simulink model "mdaq_vipstab"  (R2024b)
settings: Solver=FixedStepDiscrete  StartTime=0.0  StopTime=10  RelTol=1e-3  EnableMultiTasking=on
PreLoadFcn:
  | template_orig = fliplr([109 100]);
  | template_size = fliplr([18 22]);
  | search_border = fliplr([10 15]);
  | pos.template_orig = fliplr(template_orig);
  | pos.template_size = template_size;
  | pos.search_border = search_border;
  | pos.template_center = floor((template_size-1)/2);
  | pos.template_center_pos = pos.template_orig + ...
  |     pos.template_center - 1;
libraries: visionanalysis x1, visiongeotforms x1
settings Model: Tag="0  0  0  0  0  1"  CodeVerificationMode=processor-in-the-loop (pil)  Creator=The MathWorks Inc.  LastModifiedBy=benia
settings SolverCC: AlgebraicLoopSolver=TrustRegion
settings DataIOCC: LimitDataPoints=on  SaveFormat=Array  SignalLoggingSaveFormat=ModelDataLogs  SaveOutput=off  SaveTime=off  ReturnWorkspaceOutputs=off  SignalLoggingName=logsOut
settings OptimizationCC: DefaultParameterBehavior=Inlined  ExpressionDepthLimit=2147483647  InitFltsAndDblsToZero=on  LifeSpan=Inf  BufferReusableBoundary=off  EfficientTunableParamExpr=on
settings DebuggingCC: UnderspecifiedInitializationDetection=Classic  MergeDetectMultiDrivingBlocksExec=none  CheckExecutionContextPreStartOutputMsg=on  InheritedTsInSrcMsg=none  MultiTaskDSMMsg=warning  SigSpecEnsureSampleTimeMsg=none  ParameterPrecisionLossMsg=none  UnderSpecifiedDataTypeMsg=error  FcnCallInpInsideContextMsg=warning  UnconnectedInputMsg=warning  UnconnectedOutputMsg=warning  UnconnectedLineMsg=warning  BusObjectLabelMismatch=none  StateNameClashWarn=warning  SFUnexpectedBacktrackingDiag=warning  SFNoUnconditionalDefaultTransitionDiag=warning  SFExecutionAtInitializationDiag=none  ArithmeticOperatorsInVariantConditions=warning
settings HardwareCC: ProdBitPerLong=40  ProdBitPerPointer=32  ProdBitPerSizeT=32  ProdBitPerPtrDiffT=32  ProdLargestAtomicInteger=Integer  ProdLargestAtomicFloat=None  ProdWordSize=32  ProdHWDeviceType=Texas Instruments->C6000  TargetBitPerLong=64  TargetBitPerPointer=64  TargetBitPerSizeT=64  TargetBitPerPtrDiffT=64  TargetLongLongMode=on  TargetIntDivRoundTo=Zero  TargetEndianess=LittleEndian  TargetWordSize=64  TargetHWDeviceType=MATLAB Host
settings ModelReferenceCC: UpdateModelReferenceTargets=IfOutOfDate  PropagateSignalLabelsOutOfModel=off
settings SFSimCC: SimUseLocalCustomCode=off  MATLABDynamicMemAlloc=off  CustomCodeUndefinedFunction=UseInterfaceOnly
settings RTWCC: Description=MicroDAQ Real-Time Measurement System  SystemTargetFile=microdaq.tlc  TemplateMakefile=microdaq.tmf  PostCodeGenCommand=microdaq_postcodegen(buildInfo)  GenerateReport=on  RTWUseLocalCustomCode=off  IncludeHyperlinkInReport=on  GenerateCodeReplacementReport=on  GPUComputeCapability=3.5
settings CodeAppCC: IgnoreCustomStorageClasses=off  StateflowObjectComments=on
settings STFCustomTargetCC: CombineOutputUpdateFcns=on  ERTCustomFileBanners=on  SupportContinuousTime=off  SupportNonInlinedSFcns=off  RemoveResetFunc=on  MATLABClassNameForMDSCustomization=Simulink.SoftwareTarget.ERTCustomization  SystemTargetFile=microdaq.tlc
settings ERTTargetCC: MultiwordLength=2048  ParMdlRefBuildCompliant=off  CompOptLevelCompliant=off  ConcurrentExecutionCompliant=off  ModelStepFunctionPrototypeControlCompliant=off  CPPClassGenCompliant=off  UseToolchainInfoCompliant=off  ERTCustomFileTemplate=microdaq_main.tlc  ConvertIfToSwitch=off  SuppressUnreachableDefaultCases=off  DynamicArrayContainerType=coder::array
settings ConfigComp: CovMetricSettings=dw  CovSaveCumulativeToWorkspaceVar=on  CovSaveSingleToWorkspaceVar=on  CovExternalEMLEnable=off

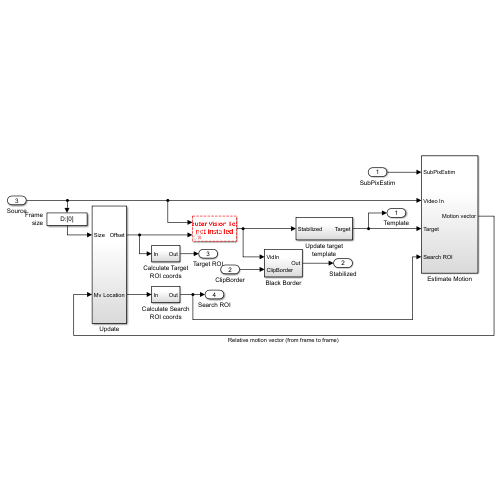
[thumbnail: Simulink's stored preview of the top-level diagram]
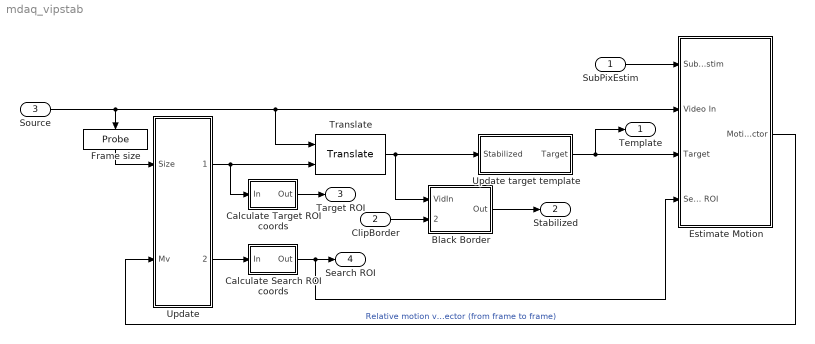
== system mdaq_vipstab ==
  SubPixEstim : Inport  OutDataTypeStr=boolean  PortDimensions=[1 1]  SampleTime=[0.033333299999999996,0]
  ClipBorder : Inport  Port=2  OutDataTypeStr=boolean  PortDimensions=[1 1]  SampleTime=[0.033333299999999996,0]
  Source : Inport  Port=3  OutDataTypeStr=uint8  PortDimensions=[320 240]  SampleTime=[0.033333299999999996,0]
  Black Border : Subsystem
  Calculate Search ROI coords : Subsystem
  Calculate Target ROI coords : Subsystem
  Estimate Motion : Subsystem
  Frame size : Probe  ProbeWidth=off  ProbeSampleTime=off  ProbeComplexSignal=off  ProbeSignalDimensions=on  ProbeDimensionsDataType=int16
  Translate : visiongeotforms/Translate  outSizeT=Same as input image  src_trans=Input port  translation="[1.5  2.3]"  maxOffset=[8 10]  fillVal=0  interpMethod=Bilinear  roundingMode=Floor  overflowMode=off  firstCoeffMode=Binary point scaling  firstCoeffWordLength=16  firstCoeffFracLength=6  prodOutputMode=Binary point scaling  prodOutputWordLength=32  prodOutputFracLength=20
  Update : Subsystem
  Update target template : Subsystem
  Template : Outport  OutDataTypeStr=uint8  PortDimensions=[22 18]  SampleTime=[0.033333299999999996,0]
  Stabilized : Outport  Port=2  OutDataTypeStr=uint8  PortDimensions=[320 240]  SampleTime=[0.033333299999999996,0]
  Target ROI : Outport  Port=3  OutDataTypeStr=fixdt('sfix16_En6')  PortDimensions=[1 4]  SampleTime=[0.033333299999999996,0]
  Search ROI : Outport  Port=4  OutDataTypeStr=fixdt('sfix16_En6')  PortDimensions=[1 4]  SampleTime=[0.033333299999999996,0]
  wires:
  Update/1(Offset) -> Calculate Target ROI coords/1(In), Translate/2
  Update/2(Location) -> Calculate Search ROI coords/1(In)
  Update target template/1(Target) -> Estimate Motion/3(Target), Template/1
  Source/1 -> Frame size/1, Estimate Motion/2(Video In), Translate/1
  Translate/1 -> Black Border/1(VidIn), Update target template/1(Stabilized)
  Estimate Motion/1(Motion vector) -> Update/2(Mv)  "Relative motion vector (from frame to frame)"
  Frame size/1 -> Update/1(Size)
  SubPixEstim/1 -> Estimate Motion/1(SubPixEstim)
  Black Border/1(Out) -> Stabilized/1
  ClipBorder/1 -> Black Border/2(ClipBorder)
  Calculate Search ROI coords/1(Out) -> Estimate Motion/4(Search ROI), Search ROI/1
  Calculate Target ROI coords/1(Out) -> Target ROI/1

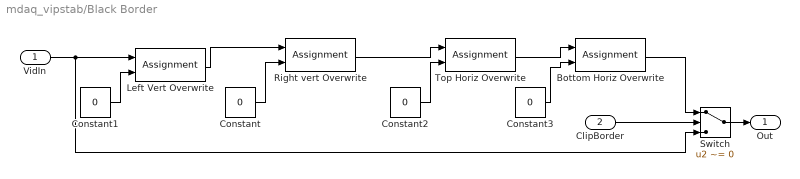
== system mdaq_vipstab/Black Border ==
  VidIn : Inport
  ClipBorder : Inport  Port=2
  Bottom Horiz Overwrite : Assignment  NumberOfDimensions=2  IndexOptions=Index vector (dialog),Assign all  Indices=[320-(pos.search_border(2)+4):320],[320-(pos.search_border(2)+4):320]  OutputSizes=1,1
  Constant{,1..3} (4 alike) : Constant  Value=0  OutDataTypeStr=uint8
  Left Vert Overwrite : Assignment  NumberOfDimensions=2  IndexOptions=Assign all,Index vector (dialog)  Indices=1:end,1:(pos.search_border(2)+4)  OutputSizes=1,1
  Right vert Overwrite : Assignment  NumberOfDimensions=2  IndexOptions=Assign all,Index vector (dialog)  Indices=1:end,[240-(pos.search_border(2)+4):240]  OutputSizes=1,1
  Switch : Switch  Criteria=u2 ~= 0  ZeroCross=off  SaturateOnIntegerOverflow=off  InputSameDT=off
  Top Horiz Overwrite : Assignment  NumberOfDimensions=2  IndexOptions=Index vector (dialog),Assign all  Indices=[1:pos.search_border(1)+4],[320-(pos.search_border(2)+4):320]  OutputSizes=1,1
  Out : Outport
  wires:
  Constant3/1 -> Bottom Horiz Overwrite/2
  Constant2/1 -> Top Horiz Overwrite/2
  Constant/1 -> Right vert Overwrite/2
  Constant1/1 -> Left Vert Overwrite/2
  Switch/1 -> Out/1
  Bottom Horiz Overwrite/1 -> Switch/1
  ClipBorder/1 -> Switch/2
  Top Horiz Overwrite/1 -> Bottom Horiz Overwrite/1
  Right vert Overwrite/1 -> Top Horiz Overwrite/1
  Left Vert Overwrite/1 -> Right vert Overwrite/1
  VidIn/1 -> Left Vert Overwrite/1, Switch/3

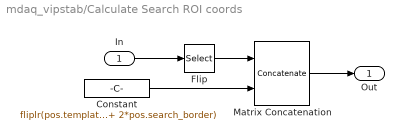
== system mdaq_vipstab/Calculate Search ROI coords ==
  In : Inport
  Constant : Constant  Value=fliplr(pos.template_size + 2*pos.search_border)  VectorParams1D=off  OutDataTypeStr=fixdt(1,16,6)
  Flip : Selector  NumberOfDimensions=2  IndexOptions=Index vector (dialog),Index vector (dialog)  Indices=1,[2 1]  OutputSizes=1,1
  Matrix Concatenation : Concatenate  Mode=Multidimensional array  ConcatenateDimension=2
  Out : Outport
  wires:
  Matrix Concatenation/1 -> Out/1
  Constant/1 -> Matrix Concatenation/2
  In/1 -> Flip/1
  Flip/1 -> Matrix Concatenation/1

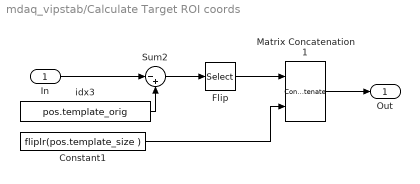
== system mdaq_vipstab/Calculate Target ROI coords ==
  In : Inport
  Constant1 : Constant  Value=fliplr(pos.template_size )  VectorParams1D=off  OutDataTypeStr=Inherit: Inherit via back propagation
  Flip : Selector  NumberOfDimensions=2  IndexOptions=Index vector (dialog),Index vector (dialog)  Indices=1,[2 1]  OutputSizes=1,1
  Matrix Concatenation1 : Concatenate  Mode=Multidimensional array  ConcatenateDimension=2
  Sum2 : Sum  Inputs=|-+
  idx3 : Constant  Value=pos.template_orig  VectorParams1D=off  OutDataTypeStr=fixdt(1,16,6)
  Out : Outport
  wires:
  idx3/1 -> Sum2/2
  Sum2/1 -> Flip/1
  Constant1/1 -> Matrix Concatenation1/2
  In/1 -> Sum2/1
  Matrix Concatenation1/1 -> Out/1
  Flip/1 -> Matrix Concatenation1/1

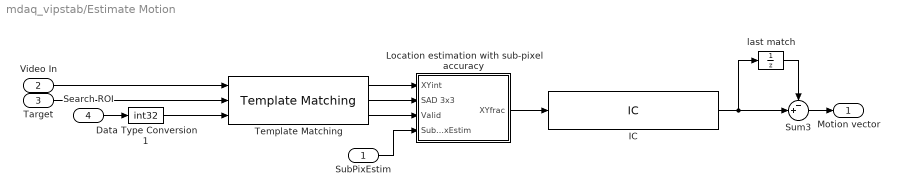
== system mdaq_vipstab/Estimate Motion ==
  SubPixEstim : Inport
  Video In : Inport  Port=2
  Target : Inport  Port=3
  Search ROI : Inport  Port=4
  Data Type Conversion1 : DataTypeConversion  OutDataTypeStr=int32  SaturateOnIntegerOverflow=off
  IC : InitialCondition  Value=fliplr(pos.template_center_pos)
  Location estimation with sub-pixel accuracy : Subsystem
  Sum3 : Sum  Inputs=-+|  OutDataTypeStr=fixdt(1,16,6)
  Template Matching : visionanalysis/Template Matching  metric=Sum of absolute differences  output=Best match location  method=Exhaustive  nMetric=on  nSize=3  roi=on  roiValid=off  roundingMode=Floor  overflowMode=off  prodOutputMode=Binary point scaling  prodOutputWordLength=32  prodOutputFracLength=0  accumMode=Binary point scaling  accumWordLength=16  accumFracLength=-2  outputMode=Binary point scaling  outputWordLength=16  outputFracLength=-2
  last match : UnitDelay  InitialCondition=fliplr(pos.template_center_pos)  SampleTime=-1  HasFrameUpgradeWarning=on
  Motion vector : Outport
  wires:
  last match/1 -> Sum3/1
  IC/1 -> last match/1, Sum3/2
  Location estimation with sub-pixel accuracy/1(XYfrac) -> IC/1
  Data Type Conversion1/1 -> Template Matching/3
  Search ROI/1 -> Data Type Conversion1/1
  SubPixEstim/1 -> Location estimation with sub-pixel accuracy/4(SubPixEstim)
  Video In/1 -> Template Matching/1
  Template Matching/3 -> Location estimation with sub-pixel accuracy/3(Valid)
  Template Matching/2 -> Location estimation with sub-pixel accuracy/2(SAD 3x3)
  Template Matching/1 -> Location estimation with sub-pixel accuracy/1(XYint)
  Target/1 -> Template Matching/2
  Sum3/1 -> Motion vector/1

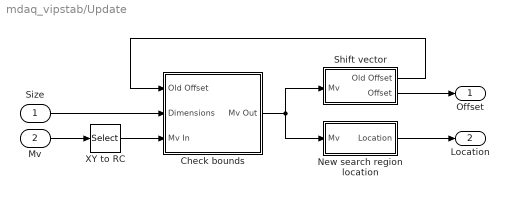
== system mdaq_vipstab/Update ==
  Size : Inport
  Mv : Inport  Port=2
  Check bounds : Subsystem
  New search region location : Subsystem
  Shift vector : Subsystem
  XY to RC : Selector  NumberOfDimensions=2  IndexOptions=Index vector (dialog),Index vector (dialog)  Indices=1,[2 1]  OutputSizes=1,1
  Offset : Outport
  Location : Outport  Port=2
  wires:
  XY to RC/1 -> Check bounds/3(Mv In)
  Check bounds/1(Mv Out) -> New search region location/1(Mv), Shift vector/1(Mv)
  Size/1 -> Check bounds/2(Dimensions)
  Shift vector/2(Offset) -> Offset/1
  New search region location/1(Location) -> Location/1
  Mv/1 -> XY to RC/1
  Shift vector/1(Old Offset) -> Check bounds/1(Old Offset)

== system mdaq_vipstab/Update target template ==
  note: cut out new template
  Stabilized : Inport
  Delay : UnitDelay  SampleTime=-1  HasFrameUpgradeWarning=on
  Selector : Selector  NumberOfDimensions=2  InputPortWidth=3  IndexOptions=Index vector (dialog),Index vector (dialog)  Indices=pos.template_orig(1)-1 : pos.template_orig(1)+pos.template_size(1)-2,pos.template_orig(2)-1 : pos.template_orig(2)+pos.template_size(2)-2  OutputSizes=1,1
  Target : Outport
  wires:
  Selector/1 -> Delay/1
  Stabilized/1 -> Selector/1
  Delay/1 -> Target/1

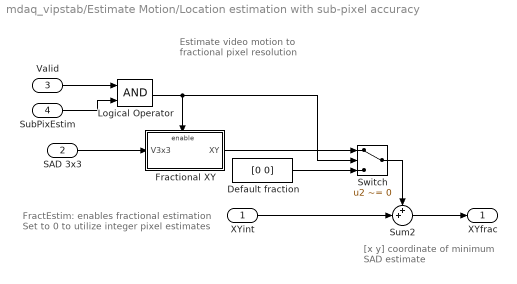
== system mdaq_vipstab/Estimate Motion/Location estimation with sub-pixel accuracy ==
  note: Estimate video motion to
      | fractional pixel resolution
  note: FractEstim: enables fractional estimation
      | Set to 0 to utilize integer pixel estimates
  note: [x y] coordinate of
      | minimum SAD estimate
  XYint : Inport
  SAD 3x3 : Inport  Port=2
  Valid : Inport  Port=3
  SubPixEstim : Inport  Port=4
  Default fraction : Constant  Value=[0 0]  VectorParams1D=off  OutDataTypeStr=fixdt(1,8,6)
  Fractional XY : Subsystem  TreatAsAtomicUnit=on
  Logical Operator : Logic  AllPortsSameDT=off  OutDataTypeStr=boolean
  Sum2 : Sum  Inputs=++|  OutDataTypeStr=fixdt(1,16,6)
  Switch : Switch  Criteria=u2 ~= 0  SaturateOnIntegerOverflow=off  InputSameDT=off
  XYfrac : Outport
  wires:
  SubPixEstim/1 -> Logical Operator/2
  Valid/1 -> Logical Operator/1
  Logical Operator/1 -> Fractional XY/Enable, Switch/2
  SAD 3x3/1 -> Fractional XY/1(V3x3)
  Sum2/1 -> XYfrac/1
  Default fraction/1 -> Switch/3
  Switch/1 -> Sum2/1
  Fractional XY/1(XY) -> Switch/1
  XYint/1 -> Sum2/2

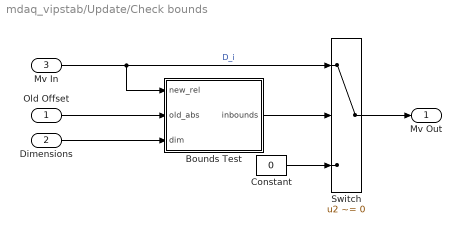
== system mdaq_vipstab/Update/Check bounds ==
  Old Offset : Inport
  Dimensions : Inport  Port=2
  Mv In : Inport  Port=3
  Bounds Test : Subsystem
  Constant : Constant  Value=0  OutDataTypeStr=fixdt(1,16,6)
  Switch : Switch  Criteria=u2 ~= 0  ZeroCross=off  SaturateOnIntegerOverflow=off  InputSameDT=off
  Mv Out : Outport
  wires:
  Old Offset/1 -> Bounds Test/2(old_abs)
  Bounds Test/1(inbounds) -> Switch/2
  Constant/1 -> Switch/3
  Dimensions/1 -> Bounds Test/3(dim)
  Switch/1 -> Mv Out/1
  Mv In/1 -> Switch/1, Bounds Test/1(new_rel)  "D_i"

== system mdaq_vipstab/Update/New search region location ==
  note: Predict new search region location
  note: This loop accumulates relative motion vector shifts
  Mv : Inport
  Sum2 : Sum  Inputs=++|  RndMeth=Nearest  LockScale=on
  Svi : UnitDelay  InitialCondition=pos.template_orig - pos.search_border - 1  SampleTime=-1  HasFrameUpgradeWarning=on
  Location : Outport
  wires:
  Svi/1 -> Sum2/1, Location/1  "Upper left corner of the search region"
  Sum2/1 -> Svi/1
  Mv/1 -> Sum2/2

== system mdaq_vipstab/Update/Shift vector ==
  note: this loop keeps track of the absolute shift of the target
  Mv : Inport
  Sum4 : Sum  Inputs=+-|  OutDataTypeStr=fixdt(1,16,6)
  Tvi : UnitDelay  SampleTime=-1  HasFrameUpgradeWarning=on
  Old Offset : Outport
  Offset : Outport  Port=2
  wires:
  Sum4/1 -> Tvi/1, Offset/1
  Tvi/1 -> Sum4/1, Old Offset/1
  Mv/1 -> Sum4/2

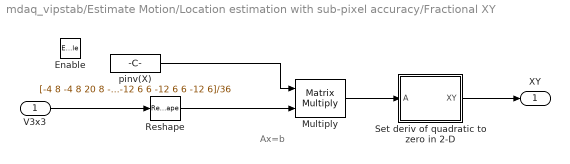
== system mdaq_vipstab/Estimate Motion/Location estimation with sub-pixel accuracy/Fractional XY ==
  note: Ax=b
  V3x3 : Inport
  Enable : EnablePort  StatesWhenEnabling=reset  PropagateVarSize=During execution  ZeroCross=off
  Multiply : Product  Inputs=**  Multiplication=Matrix(*)  OutDataTypeStr=fixdt(1,16,-1)
  Reshape : Reshape  OutputDimensionality=Column vector (2-D)
  Set deriv of quadratic to zero in 2-D : Subsystem
  pinv(X) : Constant  Value=[-4 8 -4 8 20 8 -4 8 -4;-6 -6 -6 0 0 0 6 6 6;-6 0 6 -6 0 6 -6 0 6;9 0 -9 0 0 0 -9 0 9;6 6 6 -12 -12 -12 6 6 6;6 -12 6 6 -12 6 6 -12 6]/36  VectorParams1D=off  OutDataTypeStr=fixdt(1,16)
  XY : Outport
  wires:
  Set deriv of quadratic to zero in 2-D/1(XY) -> XY/1
  Reshape/1 -> Multiply/2
  V3x3/1 -> Reshape/1
  Multiply/1 -> Set deriv of quadratic to zero in 2-D/1(A)
  pinv(X)/1 -> Multiply/1

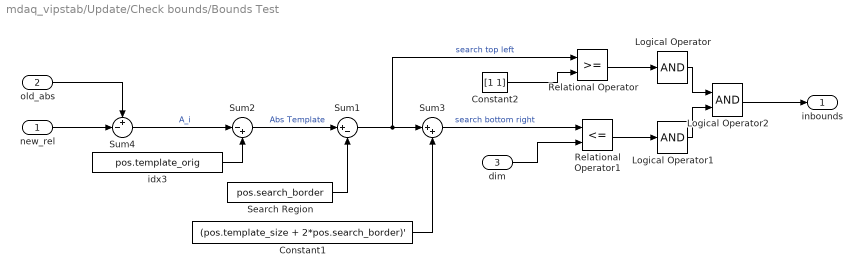
== system mdaq_vipstab/Update/Check bounds/Bounds Test ==
  new_rel : Inport
  old_abs : Inport  Port=2
  dim : Inport  Port=3
  Constant1 : Constant  Value=(pos.template_size + 2*pos.search_border)'  OutDataTypeStr=int16
  Constant2 : Constant  Value=[1 1]  OutDataTypeStr=int16
  Logical Operator : Logic  Inputs=1  AllPortsSameDT=off  OutDataTypeStr=boolean
  Logical Operator1 : Logic  Inputs=1  AllPortsSameDT=off  OutDataTypeStr=boolean
  Logical Operator2 : Logic  AllPortsSameDT=off  OutDataTypeStr=boolean
  Relational Operator : RelationalOperator  OutDataTypeStr=boolean  InputSameDT=off
  Relational Operator1 : RelationalOperator  Operator=<=  OutDataTypeStr=boolean  InputSameDT=off
  Search Region : Constant  Value=pos.search_border  OutDataTypeStr=int16
  Sum1 : Sum  Inputs=|+-  OutDataTypeStr=Inherit: Same as first input
  Sum2 : Sum  Inputs=|-+  OutDataTypeStr=int16
  Sum3 : Sum  Inputs=|++  OutDataTypeStr=Inherit: Same as first input
  Sum4 : Sum  Inputs=+-|
  idx3 : Constant  Value=pos.template_orig  OutDataTypeStr=int16
  inbounds : Outport
  wires:
  Logical Operator1/1 -> Logical Operator2/2
  Logical Operator/1 -> Logical Operator2/1
  Relational Operator/1 -> Logical Operator/1
  Relational Operator1/1 -> Logical Operator1/1
  dim/1 -> Relational Operator1/2
  Sum3/1 -> Relational Operator1/1  "search bottom right"
  Constant2/1 -> Relational Operator/2
  Constant1/1 -> Sum3/2
  Sum1/1 -> Relational Operator/1, Sum3/1  "search top left"
  Search Region/1 -> Sum1/2
  Sum2/1 -> Sum1/1  "Abs Template"
  idx3/1 -> Sum2/2
  Sum4/1 -> Sum2/1  "A_i"
  old_abs/1 -> Sum4/1
  new_rel/1 -> Sum4/2
  Logical Operator2/1 -> inbounds/1

== system mdaq_vipstab/Estimate Motion/Location estimation with sub-pixel accuracy/Fractional XY/Set deriv of quadratic to zero in 2-D ==
  A : Inport
  Matrix Concatenation : Concatenate  Mode=Multidimensional array  ConcatenateDimension=2
  x offset : Subsystem
  y offset : Subsystem
  XY : Outport
  wires:
  Matrix Concatenation/1 -> XY/1
  x offset/2(denominator) -> y offset/2(input1)
  A/1 -> y offset/1(input), x offset/1(input)
  y offset/1(output) -> Matrix Concatenation/2
  x offset/1(output) -> Matrix Concatenation/1

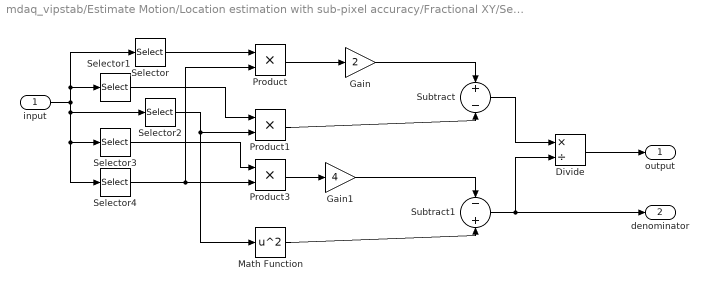
== system mdaq_vipstab/Estimate Motion/Location estimation with sub-pixel accuracy/Fractional XY/Set deriv of quadratic to zero in 2-D/x offset ==
  input : Inport
  Divide : Product  Inputs=*/  OutDataTypeStr=fixdt(1,8,6)  SaturateOnIntegerOverflow=on
  Gain : Gain  Gain=2  OutDataTypeStr=Inherit: Same as input
  Gain1 : Gain  Gain=4  OutDataTypeStr=Inherit: Same as input
  Math Function : Math  Operator=square  SignedPower=on  OutDataTypeStr=Inherit: Inherit via internal rule
  Product : Product  RndMeth=Zero
  Product1 : Product  RndMeth=Zero
  Product3 : Product  RndMeth=Zero
  Selector : Selector  IndexMode=Zero-based  IndexOptions=Index vector (dialog)  Indices=(1)  OutputSizes=1
  Selector1 : Selector  IndexMode=Zero-based  IndexOptions=Index vector (dialog)  Indices=(2)  OutputSizes=1
  Selector2 : Selector  IndexMode=Zero-based  IndexOptions=Index vector (dialog)  Indices=(3)  OutputSizes=1
  Selector3 : Selector  IndexMode=Zero-based  IndexOptions=Index vector (dialog)  Indices=(4)  OutputSizes=1
  Selector4 : Selector  IndexMode=Zero-based  IndexOptions=Index vector (dialog)  Indices=(5)  OutputSizes=1
  Subtract : Sum  Inputs=+-  OutDataTypeStr=Inherit: Same as first input
  Subtract1 : Sum  Inputs=-+  OutDataTypeStr=Inherit: Same as first input
  output : Outport
  denominator : Outport  Port=2
  wires:
  Selector4/1 -> Product3/2, Product/2
  Selector3/1 -> Product3/1
  Selector2/1 -> Math Function/1, Product1/2
  Selector1/1 -> Product1/1
  Selector/1 -> Product/1
  Math Function/1 -> Subtract1/2
  input/1 -> Selector4/1, Selector3/1, Selector2/1, Selector1/1, Selector/1
  Subtract1/1 -> denominator/1, Divide/2
  Subtract/1 -> Divide/1
  Gain1/1 -> Subtract1/1
  Product3/1 -> Gain1/1
  Product1/1 -> Subtract/2
  Gain/1 -> Subtract/1
  Product/1 -> Gain/1
  Divide/1 -> output/1

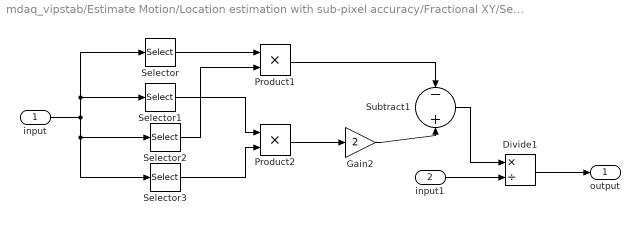
== system mdaq_vipstab/Estimate Motion/Location estimation with sub-pixel accuracy/Fractional XY/Set deriv of quadratic to zero in 2-D/y offset ==
  input : Inport
  input1 : Inport  Port=2
  Divide1 : Product  Inputs=*/  OutDataTypeStr=fixdt(1,8,6)  SaturateOnIntegerOverflow=on
  Gain2 : Gain  Gain=2  OutDataTypeStr=Inherit: Same as input
  Product1 : Product  RndMeth=Zero
  Product2 : Product  RndMeth=Zero
  Selector : Selector  IndexMode=Zero-based  IndexOptions=Index vector (dialog)  Indices=(1)  OutputSizes=1
  Selector1 : Selector  IndexMode=Zero-based  IndexOptions=Index vector (dialog)  Indices=(2)  OutputSizes=1
  Selector2 : Selector  IndexMode=Zero-based  IndexOptions=Index vector (dialog)  Indices=(3)  OutputSizes=1
  Selector3 : Selector  IndexMode=Zero-based  IndexOptions=Index vector (dialog)  Indices=(4)  OutputSizes=1
  Subtract1 : Sum  Inputs=-+
  output : Outport
  wires:
  Selector3/1 -> Product2/2
  Selector2/1 -> Product1/2
  Selector1/1 -> Product2/1
  Selector/1 -> Product1/1
  input/1 -> Selector3/1, Selector2/1, Selector1/1, Selector/1
  Product1/1 -> Subtract1/1
  Subtract1/1 -> Divide1/1
  input1/1 -> Divide1/2
  Divide1/1 -> output/1
  Product2/1 -> Gain2/1
  Gain2/1 -> Subtract1/2
